simulink model "FaceDet_x4"  (Simulink 7.7)
settings: Solver=FixedStepDiscrete  StartTime=0  StopTime=10  RelTol=1e-3
libraries: simulink x257
(part 4 of 5)

== system FaceDet_x4/FaceDetection/FU/FeatureCalcMachine3/CalcFeatureVal ==
  note: Feature can't be bigger
      | than sfix18!!!
  Lines24x15 : Inport
  LineIdxs : Inport  Port=2
  NodeWeights : Inport  Port=3
  Add : Sum  OutDataTypeStr=sint(18)
  Conv0_s3 : DataTypeConversion  OutDataTypeStr=sint(3)
  Conv0_u8 : DataTypeConversion  OutDataTypeStr=uint8
  Conv1_s3 : DataTypeConversion  OutDataTypeStr=sint(3)
  Conv1_u8 : DataTypeConversion  OutDataTypeStr=uint8
  Conv2_s3 : DataTypeConversion  OutDataTypeStr=sint(3)
  Conv2_u8 : DataTypeConversion  OutDataTypeStr=uint8
  Conv3_s3 : DataTypeConversion  OutDataTypeStr=sint(3)
  Conv3_u8 : DataTypeConversion  OutDataTypeStr=uint8
  DivideBy4 : simulink/Logic and Bit Operations/Extract Bits  SystemSampleTime=-1  bitsToExtract=Range of bits  numBits=8  bitIdxRange=[0 17]  outScalingMode=Treat bit field as an integer
  FeatureAdder : Sum  Inputs=++++  OutDataTypeStr=sint(20)
  LineIdxDemux : Demux
  NodeWeightsDemux : Demux
  ProdWgt{0..3} (4 alike) : Product  OutDataTypeStr=sint(18)  RndMeth=Zero
  SelectLine{0..3} (4 alike) : Selector  IndexMode=Zero-based  IndexOptions=Index vector (port)  Indices=1  OutputSizes=1
  ColFeatureVal : Outport
  wires:
  ProdWgt0/1 -> FeatureAdder/1
  ProdWgt1/1 -> FeatureAdder/2
  Add/1 -> FeatureAdder/3
  ProdWgt3/1 -> FeatureAdder/4
  FeatureAdder/1 -> DivideBy4/1
  LineIdxDemux/1 -> Conv0_u8/1
  Conv0_u8/1 -> SelectLine0/2
  SelectLine0/1 -> ProdWgt0/1
  LineIdxDemux/2 -> Conv1_u8/1
  Conv1_u8/1 -> SelectLine1/2
  SelectLine1/1 -> ProdWgt1/1
  Conv2_u8/1 -> SelectLine2/2
  SelectLine2/1 -> ProdWgt2/1, Add/1
  LineIdxDemux/4 -> Conv3_u8/1
  Conv3_u8/1 -> SelectLine3/2
  SelectLine3/1 -> ProdWgt3/1
  Lines24x15/1 -> SelectLine2/1, SelectLine3/1, SelectLine1/1, SelectLine0/1
  LineIdxs/1 -> LineIdxDemux/1
  LineIdxDemux/3 -> Conv2_u8/1
  NodeWeights/1 -> NodeWeightsDemux/1
  NodeWeightsDemux/4 -> Conv3_s3/1
  NodeWeightsDemux/3 -> Conv2_s3/1
  NodeWeightsDemux/2 -> Conv1_s3/1
  NodeWeightsDemux/1 -> Conv0_s3/1
  Conv3_s3/1 -> ProdWgt3/2
  DivideBy4/1 -> ColFeatureVal/1
  Conv0_s3/1 -> ProdWgt0/2
  Conv1_s3/1 -> ProdWgt1/2
  Conv2_s3/1 -> ProdWgt2/2
  ProdWgt2/1 -> Add/2

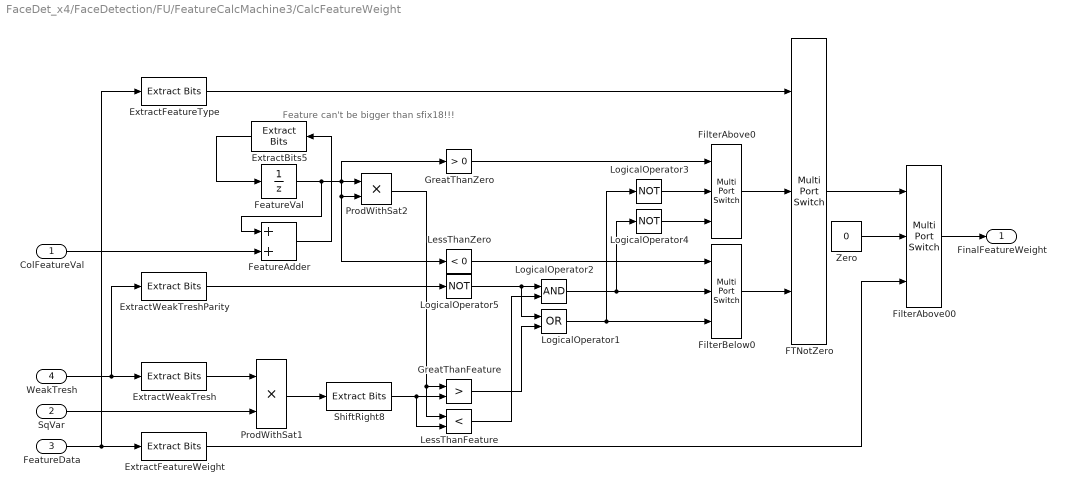
== system FaceDet_x4/FaceDetection/FU/FeatureCalcMachine3/CalcFeatureWeight ==
  note: Feature can't be bigger
      | than sfix18!!!
  ColFeatureVal : Inport
  SqVar : Inport  Port=2
  FeatureData : Inport  Port=3
  WeakTresh : Inport  Port=4
  ExtractBits5 : simulink/Logic and Bit Operations/Extract Bits  SystemSampleTime=-1  bitsToExtract=Range of bits  numBits=8  bitIdxRange=[0 17]  outScalingMode=Treat bit field as an integer
  ExtractFeatureType : simulink/Logic and Bit Operations/Extract Bits  SystemSampleTime=-1  bitsToExtract=Range of bits  numBits=8  bitIdxRange=[0 0]  outScalingMode=Treat bit field as an integer
  ExtractFeatureWeight : simulink/Logic and Bit Operations/Extract Bits  SystemSampleTime=-1  bitsToExtract=Range of bits  numBits=8  bitIdxRange=[1 16]  outScalingMode=Treat bit field as an integer
  ExtractWeakTresh : simulink/Logic and Bit Operations/Extract Bits  SystemSampleTime=-1  bitsToExtract=Range of bits  numBits=8  bitIdxRange=[1 24]  outScalingMode=Treat bit field as an integer
  ExtractWeakTreshParity : simulink/Logic and Bit Operations/Extract Bits  SystemSampleTime=-1  bitsToExtract=Range of bits  numBits=8  bitIdxRange=[0 0]  outScalingMode=Treat bit field as an integer
  FTNotZero : MultiPortSwitch  DataPortOrder=Zero-based contiguous  Inputs=2  zeroidx=on
  FeatureAdder : Sum  OutDataTypeStr=sint(19)
  FeatureVal : UnitDelay
  FilterAbove0 : MultiPortSwitch  DataPortOrder=Zero-based contiguous  Inputs=2  zeroidx=on
  FilterAbove00 : MultiPortSwitch  DataPortOrder=Zero-based contiguous  Inputs=2  zeroidx=on
  FilterBelow0 : MultiPortSwitch  DataPortOrder=Zero-based contiguous  Inputs=2  zeroidx=on
  GreatThanFeature : RelationalOperator  Operator=>  OutDataTypeStr=boolean
  GreatThanZero : simulink/Logic and Bit Operations/Compare To Zero  SystemSampleTime=-1  relop=>  LogicOutDataTypeMode=boolean  ZeroCross=off
  LessThanFeature : RelationalOperator  Operator=<  OutDataTypeStr=boolean
  LessThanZero : simulink/Logic and Bit Operations/Compare To Zero  SystemSampleTime=-1  relop=<  LogicOutDataTypeMode=boolean  ZeroCross=off
  LogicalOperator1 : Logic  Operator=OR  AllPortsSameDT=off  OutDataTypeStr=boolean
  LogicalOperator2 : Logic  AllPortsSameDT=off  OutDataTypeStr=boolean
  LogicalOperator3 : Logic  Operator=NOT  AllPortsSameDT=off  OutDataTypeStr=boolean
  LogicalOperator4 : Logic  Operator=NOT  AllPortsSameDT=off  OutDataTypeStr=boolean
  LogicalOperator5 : Logic  Operator=NOT  AllPortsSameDT=off  OutDataTypeStr=boolean
  ProdWithSat1 : Product  OutDataTypeStr=uint(32)  SaturateOnIntegerOverflow=on  RndMeth=Zero
  ProdWithSat2 : Product  OutDataTypeStr=uint32  SaturateOnIntegerOverflow=on  RndMeth=Zero
  ShiftRight8 : simulink/Logic and Bit Operations/Extract Bits  SystemSampleTime=-1  bitsToExtract=Range of bits  numBits=8  bitIdxRange=[8 31]  outScalingMode=Treat bit field as an integer
  Zero : Constant  Value=0  OutDataTypeStr=uint16
  FinalFeatureWeight : Outport
  wires:
  FeatureVal/1 -> FeatureAdder/1, GreatThanZero/1, ProdWithSat2/1, LessThanZero/1, ProdWithSat2/2
  FeatureAdder/1 -> ExtractBits5/1
  ProdWithSat2/1 -> GreatThanFeature/1, LessThanFeature/1
  LogicalOperator4/1 -> FilterAbove0/3
  ShiftRight8/1 -> LessThanFeature/2, GreatThanFeature/2
  ProdWithSat1/1 -> ShiftRight8/1
  FilterBelow0/1 -> FTNotZero/3
  FilterAbove0/1 -> FTNotZero/2
  LogicalOperator3/1 -> FilterAbove0/2
  GreatThanZero/1 -> FilterAbove0/1
  LessThanZero/1 -> FilterBelow0/1
  Zero/1 -> FilterAbove00/2
  FTNotZero/1 -> FilterAbove00/1
  LogicalOperator5/1 -> LogicalOperator2/1, LogicalOperator1/1
  LessThanFeature/1 -> LogicalOperator2/2
  LogicalOperator2/1 -> LogicalOperator4/1, FilterBelow0/2
  LogicalOperator1/1 -> LogicalOperator3/1, FilterBelow0/3
  GreatThanFeature/1 -> LogicalOperator1/2
  WeakTresh/1 -> ExtractWeakTresh/1, ExtractWeakTreshParity/1
  SqVar/1 -> ProdWithSat1/2
  FeatureData/1 -> ExtractFeatureWeight/1, ExtractFeatureType/1
  FilterAbove00/1 -> FinalFeatureWeight/1
  ColFeatureVal/1 -> FeatureAdder/2
  ExtractBits5/1 -> FeatureVal/1
  ExtractFeatureWeight/1 -> FilterAbove00/3
  ExtractFeatureType/1 -> FTNotZero/1
  ExtractWeakTresh/1 -> ProdWithSat1/1
  ExtractWeakTreshParity/1 -> LogicalOperator5/1

== system FaceDet_x4/FaceDetection/FU/MemBank/FeatureDataMem ==
  FeatureDataLatch : Inport
  FeatureDataExt : Inport  Port=2
  Comb4FeatureData : Mux
  FeatureData{0..3} (4 alike) : simulink/Additional Math & Discrete/Additional Discrete/Unit Delay Enabled  SystemSampleTime=-1  vinit=0  tsamp=-1
  FeatureData : Outport
  wires:
  FeatureDataExt/1 -> FeatureData0/1, FeatureData1/1, FeatureData2/1, FeatureData3/1
  FeatureData0/1 -> Comb4FeatureData/1
  FeatureDataLatch/1 -> FeatureData0/2, FeatureData1/2, FeatureData2/2, FeatureData3/2
  Comb4FeatureData/1 -> FeatureData/1
  FeatureData1/1 -> Comb4FeatureData/2
  FeatureData2/1 -> Comb4FeatureData/3
  FeatureData3/1 -> Comb4FeatureData/4

== system FaceDet_x4/FaceDetection/FU/MemBank/LineIdxsMem ==
  LineIdxsLatch : Inport
  LineIdxsExt : Inport  Port=2
  Comb4LineIdxs : Mux
  LineIdxsBank{0..3} (4 alike) : simulink/Additional Math & Discrete/Additional Discrete/Unit Delay Enabled  SystemSampleTime=-1  vinit=0  tsamp=-1
  LineIdxs : Outport
  wires:
  Comb4LineIdxs/1 -> LineIdxs/1
  LineIdxsLatch/1 -> LineIdxsBank0/2, LineIdxsBank1/2, LineIdxsBank2/2, LineIdxsBank3/2
  LineIdxsBank0/1 -> Comb4LineIdxs/1
  LineIdxsExt/1 -> LineIdxsBank0/1, LineIdxsBank1/1, LineIdxsBank2/1, LineIdxsBank3/1
  LineIdxsBank1/1 -> Comb4LineIdxs/2
  LineIdxsBank3/1 -> Comb4LineIdxs/4
  LineIdxsBank2/1 -> Comb4LineIdxs/3

== system FaceDet_x4/FaceDetection/FU/MemBank/NodeWeightsMem ==
  NodeWeightsCtrlRdAdr : Inport
  NodeWeightsCtrlWrAdr : Inport  Port=2
  NodeWeightsCtrlEn : Inport  Port=3
  NodeWeightsExt : Inport  Port=4
  Comb4NodeWeights : Mux
  NodeWeightsBank0 : Subsystem  mask(Dual-port RAM){ram_size=5}
      mask prompts: ram_size "Address port width (2 to 16)"
      mask help:
      | This block simulates a dual-port RAM with registered address.
      |
      | The read and write address port width is limited to between 2 to 16 bits.
      mask init:
      | hdlblkmask_dpram;
      settings: ErrorFcn=hdlblkmask_errfcn
      mask Help: helpview([docroot '/toolbox/slhdlcoder/slhdlcoder_ug.map'],'HDL_dual_port_RAM');
      mask Display: disp( 'DualPortRam' )
  NodeWeightsBank1 : Subsystem  mask(Dual-port RAM){ram_size=5}
      mask prompts: ram_size "Address port width (2 to 16)"
      mask help:
      | This block simulates a dual-port RAM with registered address.
      |
      | The read and write address port width is limited to between 2 to 16 bits.
      mask init:
      | hdlblkmask_dpram;
      settings: ErrorFcn=hdlblkmask_errfcn
      mask Help: helpview([docroot '/toolbox/slhdlcoder/slhdlcoder_ug.map'],'HDL_dual_port_RAM');
      mask Display: disp( 'DualPortRam' )
  NodeWeightsBank2 : Subsystem  mask(Dual-port RAM){ram_size=5}
      mask prompts: ram_size "Address port width (2 to 16)"
      mask help:
      | This block simulates a dual-port RAM with registered address.
      |
      | The read and write address port width is limited to between 2 to 16 bits.
      mask init:
      | hdlblkmask_dpram;
      settings: ErrorFcn=hdlblkmask_errfcn
      mask Help: helpview([docroot '/toolbox/slhdlcoder/slhdlcoder_ug.map'],'HDL_dual_port_RAM');
      mask Display: disp( 'DualPortRam' )
  NodeWeightsBank3 : Subsystem  mask(Dual-port RAM){ram_size=5}
      mask prompts: ram_size "Address port width (2 to 16)"
      mask help:
      | This block simulates a dual-port RAM with registered address.
      |
      | The read and write address port width is limited to between 2 to 16 bits.
      mask init:
      | hdlblkmask_dpram;
      settings: ErrorFcn=hdlblkmask_errfcn
      mask Help: helpview([docroot '/toolbox/slhdlcoder/slhdlcoder_ug.map'],'HDL_dual_port_RAM');
      mask Display: disp( 'DualPortRam' )
  NodeWeights : Outport
  wires:
  NodeWeightsExt/1 -> NodeWeightsBank0/2(wr_din), NodeWeightsBank2/2(wr_din), NodeWeightsBank3/2(wr_din), NodeWeightsBank1/2(wr_din)
  NodeWeightsBank3/1(rd_dout) -> Comb4NodeWeights/4
  NodeWeightsBank2/1(rd_dout) -> Comb4NodeWeights/3
  NodeWeightsBank1/1(rd_dout) -> Comb4NodeWeights/2
  NodeWeightsBank0/1(rd_dout) -> Comb4NodeWeights/1
  NodeWeightsCtrlWrAdr/1 -> NodeWeightsBank2/4(wr_addr), NodeWeightsBank3/4(wr_addr), NodeWeightsBank1/4(wr_addr), NodeWeightsBank0/4(wr_addr)
  NodeWeightsCtrlEn/1 -> NodeWeightsBank2/3(wr_en), NodeWeightsBank3/3(wr_en), NodeWeightsBank1/3(wr_en), NodeWeightsBank0/3(wr_en)
  NodeWeightsCtrlRdAdr/1 -> NodeWeightsBank2/1(rd_addr), NodeWeightsBank3/1(rd_addr), NodeWeightsBank1/1(rd_addr), NodeWeightsBank0/1(rd_addr)
  Comb4NodeWeights/1 -> NodeWeights/1

== system FaceDet_x4/FaceDetection/FU/MemBank/WeakTreshMem ==
  WeakTreshLatch : Inport
  WeakTreshExt : Inport  Port=2
  Comb4WeakTresh : Mux
  WeakTresh{0..3} (4 alike) : simulink/Additional Math & Discrete/Additional Discrete/Unit Delay Enabled  SystemSampleTime=-1  vinit=0  tsamp=-1
  WeakTresh : Outport
  wires:
  WeakTresh3/1 -> Comb4WeakTresh/4
  WeakTresh2/1 -> Comb4WeakTresh/3
  WeakTresh1/1 -> Comb4WeakTresh/2
  Comb4WeakTresh/1 -> WeakTresh/1
  WeakTreshLatch/1 -> WeakTresh2/2, WeakTresh3/2, WeakTresh1/2, WeakTresh0/2
  WeakTresh0/1 -> Comb4WeakTresh/1
  WeakTreshExt/1 -> WeakTresh2/1, WeakTresh3/1, WeakTresh1/1, WeakTresh0/1

== system FaceDet_x4/FaceDetection/FU/CalcIntegralImg/HorzRunningSum/Accumulator0 ==
  note: AccumulatorBlock
  In : Inport
  En : Inport  Port=2
  Rst : Inport  Port=3
  Adder : Sum  OutDataTypeStr=uint(NBits)
  UDlyER : Subsystem  mask(Unit Delay Enabled Resettable){vinit=0, tsamp=-1}
      mask prompts: vinit "Initial condition:"; tsamp "Sample time:"
      mask help:
      | Normally, the output is the signal u delayed by one sample period.
      | When the reset signal R is true, the state is always set equal to the initial condition parameter.  This reset action is vectorized and supports scalar expansion.
      | When the enable signal is false, the block is disabled, and the state and output values do not change except for resets.  The enable action is vectorized and supports scalar expansion.
      mask Display: dpoly(1,[1 0],'z')
  Acc : Outport
  wires:
  En/1 -> UDlyER/2(E)
  Rst/1 -> UDlyER/3(R)
  In/1 -> Adder/1
  Adder/1 -> UDlyER/1(u), Acc/1
  UDlyER/1(y) -> Adder/2

== system FaceDet_x4/FaceDetection/FU/CalcIntegralImg/HorzRunningSum/Accumulator1 ==
  note: AccumulatorBlock
  In : Inport
  En : Inport  Port=2
  Rst : Inport  Port=3
  Adder : Sum  OutDataTypeStr=uint(NBits)
  UDlyER : Subsystem  mask(Unit Delay Enabled Resettable){vinit=0, tsamp=-1}
      mask prompts: vinit "Initial condition:"; tsamp "Sample time:"
      mask help:
      | Normally, the output is the signal u delayed by one sample period.
      | When the reset signal R is true, the state is always set equal to the initial condition parameter.  This reset action is vectorized and supports scalar expansion.
      | When the enable signal is false, the block is disabled, and the state and output values do not change except for resets.  The enable action is vectorized and supports scalar expansion.
      mask Display: dpoly(1,[1 0],'z')
  Acc : Outport
  wires:
  UDlyER/1(y) -> Adder/2
  Adder/1 -> Acc/1, UDlyER/1(u)
  In/1 -> Adder/1
  Rst/1 -> UDlyER/3(R)
  En/1 -> UDlyER/2(E)

== system FaceDet_x4/FaceDetection/FU/CalcIntegralImg/HorzRunningSum/Accumulator10 ==
  note: AccumulatorBlock
  In : Inport
  En : Inport  Port=2
  Rst : Inport  Port=3
  Adder : Sum  OutDataTypeStr=uint(NBits)
  UDlyER : Subsystem  mask(Unit Delay Enabled Resettable){vinit=0, tsamp=-1}
      mask prompts: vinit "Initial condition:"; tsamp "Sample time:"
      mask help:
      | Normally, the output is the signal u delayed by one sample period.
      | When the reset signal R is true, the state is always set equal to the initial condition parameter.  This reset action is vectorized and supports scalar expansion.
      | When the enable signal is false, the block is disabled, and the state and output values do not change except for resets.  The enable action is vectorized and supports scalar expansion.
      mask Display: dpoly(1,[1 0],'z')
  Acc : Outport
  wires:
  En/1 -> UDlyER/2(E)
  Rst/1 -> UDlyER/3(R)
  In/1 -> Adder/1
  Adder/1 -> UDlyER/1(u), Acc/1
  UDlyER/1(y) -> Adder/2

== system FaceDet_x4/FaceDetection/FU/CalcIntegralImg/HorzRunningSum/Accumulator11 ==
  note: AccumulatorBlock
  In : Inport
  En : Inport  Port=2
  Rst : Inport  Port=3
  Adder : Sum  OutDataTypeStr=uint(NBits)
  UDlyER : Subsystem  mask(Unit Delay Enabled Resettable){vinit=0, tsamp=-1}
      mask prompts: vinit "Initial condition:"; tsamp "Sample time:"
      mask help:
      | Normally, the output is the signal u delayed by one sample period.
      | When the reset signal R is true, the state is always set equal to the initial condition parameter.  This reset action is vectorized and supports scalar expansion.
      | When the enable signal is false, the block is disabled, and the state and output values do not change except for resets.  The enable action is vectorized and supports scalar expansion.
      mask Display: dpoly(1,[1 0],'z')
  Acc : Outport
  wires:
  UDlyER/1(y) -> Adder/2
  Adder/1 -> Acc/1, UDlyER/1(u)
  In/1 -> Adder/1
  Rst/1 -> UDlyER/3(R)
  En/1 -> UDlyER/2(E)

== system FaceDet_x4/FaceDetection/FU/CalcIntegralImg/HorzRunningSum/Accumulator12 ==
  note: AccumulatorBlock
  In : Inport
  En : Inport  Port=2
  Rst : Inport  Port=3
  Adder : Sum  OutDataTypeStr=uint(NBits)
  UDlyER : Subsystem  mask(Unit Delay Enabled Resettable){vinit=0, tsamp=-1}
      mask prompts: vinit "Initial condition:"; tsamp "Sample time:"
      mask help:
      | Normally, the output is the signal u delayed by one sample period.
      | When the reset signal R is true, the state is always set equal to the initial condition parameter.  This reset action is vectorized and supports scalar expansion.
      | When the enable signal is false, the block is disabled, and the state and output values do not change except for resets.  The enable action is vectorized and supports scalar expansion.
      mask Display: dpoly(1,[1 0],'z')
  Acc : Outport
  wires:
  En/1 -> UDlyER/2(E)
  Rst/1 -> UDlyER/3(R)
  In/1 -> Adder/1
  Adder/1 -> UDlyER/1(u), Acc/1
  UDlyER/1(y) -> Adder/2

== system FaceDet_x4/FaceDetection/FU/CalcIntegralImg/HorzRunningSum/Accumulator13 ==
  note: AccumulatorBlock
  In : Inport
  En : Inport  Port=2
  Rst : Inport  Port=3
  Adder : Sum  OutDataTypeStr=uint(NBits)
  UDlyER : Subsystem  mask(Unit Delay Enabled Resettable){vinit=0, tsamp=-1}
      mask prompts: vinit "Initial condition:"; tsamp "Sample time:"
      mask help:
      | Normally, the output is the signal u delayed by one sample period.
      | When the reset signal R is true, the state is always set equal to the initial condition parameter.  This reset action is vectorized and supports scalar expansion.
      | When the enable signal is false, the block is disabled, and the state and output values do not change except for resets.  The enable action is vectorized and supports scalar expansion.
      mask Display: dpoly(1,[1 0],'z')
  Acc : Outport
  wires:
  UDlyER/1(y) -> Adder/2
  Adder/1 -> Acc/1, UDlyER/1(u)
  In/1 -> Adder/1
  Rst/1 -> UDlyER/3(R)
  En/1 -> UDlyER/2(E)

== system FaceDet_x4/FaceDetection/FU/CalcIntegralImg/HorzRunningSum/Accumulator14 ==
  note: AccumulatorBlock
  In : Inport
  En : Inport  Port=2
  Rst : Inport  Port=3
  Adder : Sum  OutDataTypeStr=uint(NBits)
  UDlyER : Subsystem  mask(Unit Delay Enabled Resettable){vinit=0, tsamp=-1}
      mask prompts: vinit "Initial condition:"; tsamp "Sample time:"
      mask help:
      | Normally, the output is the signal u delayed by one sample period.
      | When the reset signal R is true, the state is always set equal to the initial condition parameter.  This reset action is vectorized and supports scalar expansion.
      | When the enable signal is false, the block is disabled, and the state and output values do not change except for resets.  The enable action is vectorized and supports scalar expansion.
      mask Display: dpoly(1,[1 0],'z')
  Acc : Outport
  wires:
  En/1 -> UDlyER/2(E)
  Rst/1 -> UDlyER/3(R)
  In/1 -> Adder/1
  Adder/1 -> UDlyER/1(u), Acc/1
  UDlyER/1(y) -> Adder/2

== system FaceDet_x4/FaceDetection/FU/CalcIntegralImg/HorzRunningSum/Accumulator15 ==
  note: AccumulatorBlock
  In : Inport
  En : Inport  Port=2
  Rst : Inport  Port=3
  Adder : Sum  OutDataTypeStr=uint(NBits)
  UDlyER : Subsystem  mask(Unit Delay Enabled Resettable){vinit=0, tsamp=-1}
      mask prompts: vinit "Initial condition:"; tsamp "Sample time:"
      mask help:
      | Normally, the output is the signal u delayed by one sample period.
      | When the reset signal R is true, the state is always set equal to the initial condition parameter.  This reset action is vectorized and supports scalar expansion.
      | When the enable signal is false, the block is disabled, and the state and output values do not change except for resets.  The enable action is vectorized and supports scalar expansion.
      mask Display: dpoly(1,[1 0],'z')
  Acc : Outport
  wires:
  UDlyER/1(y) -> Adder/2
  Adder/1 -> Acc/1, UDlyER/1(u)
  In/1 -> Adder/1
  Rst/1 -> UDlyER/3(R)
  En/1 -> UDlyER/2(E)

== system FaceDet_x4/FaceDetection/FU/CalcIntegralImg/HorzRunningSum/Accumulator16 ==
  note: AccumulatorBlock
  In : Inport
  En : Inport  Port=2
  Rst : Inport  Port=3
  Adder : Sum  OutDataTypeStr=uint(NBits)
  UDlyER : Subsystem  mask(Unit Delay Enabled Resettable){vinit=0, tsamp=-1}
      mask prompts: vinit "Initial condition:"; tsamp "Sample time:"
      mask help:
      | Normally, the output is the signal u delayed by one sample period.
      | When the reset signal R is true, the state is always set equal to the initial condition parameter.  This reset action is vectorized and supports scalar expansion.
      | When the enable signal is false, the block is disabled, and the state and output values do not change except for resets.  The enable action is vectorized and supports scalar expansion.
      mask Display: dpoly(1,[1 0],'z')
  Acc : Outport
  wires:
  En/1 -> UDlyER/2(E)
  Rst/1 -> UDlyER/3(R)
  In/1 -> Adder/1
  Adder/1 -> UDlyER/1(u), Acc/1
  UDlyER/1(y) -> Adder/2

== system FaceDet_x4/FaceDetection/FU/CalcIntegralImg/HorzRunningSum/Accumulator17 ==
  note: AccumulatorBlock
  In : Inport
  En : Inport  Port=2
  Rst : Inport  Port=3
  Adder : Sum  OutDataTypeStr=uint(NBits)
  UDlyER : Subsystem  mask(Unit Delay Enabled Resettable){vinit=0, tsamp=-1}
      mask prompts: vinit "Initial condition:"; tsamp "Sample time:"
      mask help:
      | Normally, the output is the signal u delayed by one sample period.
      | When the reset signal R is true, the state is always set equal to the initial condition parameter.  This reset action is vectorized and supports scalar expansion.
      | When the enable signal is false, the block is disabled, and the state and output values do not change except for resets.  The enable action is vectorized and supports scalar expansion.
      mask Display: dpoly(1,[1 0],'z')
  Acc : Outport
  wires:
  UDlyER/1(y) -> Adder/2
  Adder/1 -> Acc/1, UDlyER/1(u)
  In/1 -> Adder/1
  Rst/1 -> UDlyER/3(R)
  En/1 -> UDlyER/2(E)

== system FaceDet_x4/FaceDetection/FU/CalcIntegralImg/HorzRunningSum/Accumulator18 ==
  note: AccumulatorBlock
  In : Inport
  En : Inport  Port=2
  Rst : Inport  Port=3
  Adder : Sum  OutDataTypeStr=uint(NBits)
  UDlyER : Subsystem  mask(Unit Delay Enabled Resettable){vinit=0, tsamp=-1}
      mask prompts: vinit "Initial condition:"; tsamp "Sample time:"
      mask help:
      | Normally, the output is the signal u delayed by one sample period.
      | When the reset signal R is true, the state is always set equal to the initial condition parameter.  This reset action is vectorized and supports scalar expansion.
      | When the enable signal is false, the block is disabled, and the state and output values do not change except for resets.  The enable action is vectorized and supports scalar expansion.
      mask Display: dpoly(1,[1 0],'z')
  Acc : Outport
  wires:
  En/1 -> UDlyER/2(E)
  Rst/1 -> UDlyER/3(R)
  In/1 -> Adder/1
  Adder/1 -> UDlyER/1(u), Acc/1
  UDlyER/1(y) -> Adder/2

== system FaceDet_x4/FaceDetection/FU/CalcIntegralImg/HorzRunningSum/Accumulator19 ==
  note: AccumulatorBlock
  In : Inport
  En : Inport  Port=2
  Rst : Inport  Port=3
  Adder : Sum  OutDataTypeStr=uint(NBits)
  UDlyER : Subsystem  mask(Unit Delay Enabled Resettable){vinit=0, tsamp=-1}
      mask prompts: vinit "Initial condition:"; tsamp "Sample time:"
      mask help:
      | Normally, the output is the signal u delayed by one sample period.
      | When the reset signal R is true, the state is always set equal to the initial condition parameter.  This reset action is vectorized and supports scalar expansion.
      | When the enable signal is false, the block is disabled, and the state and output values do not change except for resets.  The enable action is vectorized and supports scalar expansion.
      mask Display: dpoly(1,[1 0],'z')
  Acc : Outport
  wires:
  UDlyER/1(y) -> Adder/2
  Adder/1 -> Acc/1, UDlyER/1(u)
  In/1 -> Adder/1
  Rst/1 -> UDlyER/3(R)
  En/1 -> UDlyER/2(E)

== system FaceDet_x4/FaceDetection/FU/CalcIntegralImg/HorzRunningSum/Accumulator2 ==
  note: AccumulatorBlock
  In : Inport
  En : Inport  Port=2
  Rst : Inport  Port=3
  Adder : Sum  OutDataTypeStr=uint(NBits)
  UDlyER : Subsystem  mask(Unit Delay Enabled Resettable){vinit=0, tsamp=-1}
      mask prompts: vinit "Initial condition:"; tsamp "Sample time:"
      mask help:
      | Normally, the output is the signal u delayed by one sample period.
      | When the reset signal R is true, the state is always set equal to the initial condition parameter.  This reset action is vectorized and supports scalar expansion.
      | When the enable signal is false, the block is disabled, and the state and output values do not change except for resets.  The enable action is vectorized and supports scalar expansion.
      mask Display: dpoly(1,[1 0],'z')
  Acc : Outport
  wires:
  En/1 -> UDlyER/2(E)
  Rst/1 -> UDlyER/3(R)
  In/1 -> Adder/1
  Adder/1 -> UDlyER/1(u), Acc/1
  UDlyER/1(y) -> Adder/2

== system FaceDet_x4/FaceDetection/FU/CalcIntegralImg/HorzRunningSum/Accumulator20 ==
  note: AccumulatorBlock
  In : Inport
  En : Inport  Port=2
  Rst : Inport  Port=3
  Adder : Sum  OutDataTypeStr=uint(NBits)
  UDlyER : Subsystem  mask(Unit Delay Enabled Resettable){vinit=0, tsamp=-1}
      mask prompts: vinit "Initial condition:"; tsamp "Sample time:"
      mask help:
      | Normally, the output is the signal u delayed by one sample period.
      | When the reset signal R is true, the state is always set equal to the initial condition parameter.  This reset action is vectorized and supports scalar expansion.
      | When the enable signal is false, the block is disabled, and the state and output values do not change except for resets.  The enable action is vectorized and supports scalar expansion.
      mask Display: dpoly(1,[1 0],'z')
  Acc : Outport
  wires:
  En/1 -> UDlyER/2(E)
  Rst/1 -> UDlyER/3(R)
  In/1 -> Adder/1
  Adder/1 -> UDlyER/1(u), Acc/1
  UDlyER/1(y) -> Adder/2

== system FaceDet_x4/FaceDetection/FU/CalcIntegralImg/HorzRunningSum/Accumulator21 ==
  note: AccumulatorBlock
  In : Inport
  En : Inport  Port=2
  Rst : Inport  Port=3
  Adder : Sum  OutDataTypeStr=uint(NBits)
  UDlyER : Subsystem  mask(Unit Delay Enabled Resettable){vinit=0, tsamp=-1}
      mask prompts: vinit "Initial condition:"; tsamp "Sample time:"
      mask help:
      | Normally, the output is the signal u delayed by one sample period.
      | When the reset signal R is true, the state is always set equal to the initial condition parameter.  This reset action is vectorized and supports scalar expansion.
      | When the enable signal is false, the block is disabled, and the state and output values do not change except for resets.  The enable action is vectorized and supports scalar expansion.
      mask Display: dpoly(1,[1 0],'z')
  Acc : Outport
  wires:
  UDlyER/1(y) -> Adder/2
  Adder/1 -> Acc/1, UDlyER/1(u)
  In/1 -> Adder/1
  Rst/1 -> UDlyER/3(R)
  En/1 -> UDlyER/2(E)

== system FaceDet_x4/FaceDetection/FU/CalcIntegralImg/HorzRunningSum/Accumulator22 ==
  note: AccumulatorBlock
  In : Inport
  En : Inport  Port=2
  Rst : Inport  Port=3
  Adder : Sum  OutDataTypeStr=uint(NBits)
  UDlyER : Subsystem  mask(Unit Delay Enabled Resettable){vinit=0, tsamp=-1}
      mask prompts: vinit "Initial condition:"; tsamp "Sample time:"
      mask help:
      | Normally, the output is the signal u delayed by one sample period.
      | When the reset signal R is true, the state is always set equal to the initial condition parameter.  This reset action is vectorized and supports scalar expansion.
      | When the enable signal is false, the block is disabled, and the state and output values do not change except for resets.  The enable action is vectorized and supports scalar expansion.
      mask Display: dpoly(1,[1 0],'z')
  Acc : Outport
  wires:
  En/1 -> UDlyER/2(E)
  Rst/1 -> UDlyER/3(R)
  In/1 -> Adder/1
  Adder/1 -> UDlyER/1(u), Acc/1
  UDlyER/1(y) -> Adder/2

== system FaceDet_x4/FaceDetection/FU/CalcIntegralImg/HorzRunningSum/Accumulator23 ==
  note: AccumulatorBlock
  In : Inport
  En : Inport  Port=2
  Rst : Inport  Port=3
  Adder : Sum  OutDataTypeStr=uint(NBits)
  UDlyER : Subsystem  mask(Unit Delay Enabled Resettable){vinit=0, tsamp=-1}
      mask prompts: vinit "Initial condition:"; tsamp "Sample time:"
      mask help:
      | Normally, the output is the signal u delayed by one sample period.
      | When the reset signal R is true, the state is always set equal to the initial condition parameter.  This reset action is vectorized and supports scalar expansion.
      | When the enable signal is false, the block is disabled, and the state and output values do not change except for resets.  The enable action is vectorized and supports scalar expansion.
      mask Display: dpoly(1,[1 0],'z')
  Acc : Outport
  wires:
  UDlyER/1(y) -> Adder/2
  Adder/1 -> Acc/1, UDlyER/1(u)
  In/1 -> Adder/1
  Rst/1 -> UDlyER/3(R)
  En/1 -> UDlyER/2(E)

== system FaceDet_x4/FaceDetection/FU/CalcIntegralImg/HorzRunningSum/Accumulator3 ==
  note: AccumulatorBlock
  In : Inport
  En : Inport  Port=2
  Rst : Inport  Port=3
  Adder : Sum  OutDataTypeStr=uint(NBits)
  UDlyER : Subsystem  mask(Unit Delay Enabled Resettable){vinit=0, tsamp=-1}
      mask prompts: vinit "Initial condition:"; tsamp "Sample time:"
      mask help:
      | Normally, the output is the signal u delayed by one sample period.
      | When the reset signal R is true, the state is always set equal to the initial condition parameter.  This reset action is vectorized and supports scalar expansion.
      | When the enable signal is false, the block is disabled, and the state and output values do not change except for resets.  The enable action is vectorized and supports scalar expansion.
      mask Display: dpoly(1,[1 0],'z')
  Acc : Outport
  wires:
  UDlyER/1(y) -> Adder/2
  Adder/1 -> Acc/1, UDlyER/1(u)
  In/1 -> Adder/1
  Rst/1 -> UDlyER/3(R)
  En/1 -> UDlyER/2(E)

== system FaceDet_x4/FaceDetection/FU/CalcIntegralImg/HorzRunningSum/Accumulator4 ==
  note: AccumulatorBlock
  In : Inport
  En : Inport  Port=2
  Rst : Inport  Port=3
  Adder : Sum  OutDataTypeStr=uint(NBits)
  UDlyER : Subsystem  mask(Unit Delay Enabled Resettable){vinit=0, tsamp=-1}
      mask prompts: vinit "Initial condition:"; tsamp "Sample time:"
      mask help:
      | Normally, the output is the signal u delayed by one sample period.
      | When the reset signal R is true, the state is always set equal to the initial condition parameter.  This reset action is vectorized and supports scalar expansion.
      | When the enable signal is false, the block is disabled, and the state and output values do not change except for resets.  The enable action is vectorized and supports scalar expansion.
      mask Display: dpoly(1,[1 0],'z')
  Acc : Outport
  wires:
  En/1 -> UDlyER/2(E)
  Rst/1 -> UDlyER/3(R)
  In/1 -> Adder/1
  Adder/1 -> UDlyER/1(u), Acc/1
  UDlyER/1(y) -> Adder/2

== system FaceDet_x4/FaceDetection/FU/CalcIntegralImg/HorzRunningSum/Accumulator5 ==
  note: AccumulatorBlock
  In : Inport
  En : Inport  Port=2
  Rst : Inport  Port=3
  Adder : Sum  OutDataTypeStr=uint(NBits)
  UDlyER : Subsystem  mask(Unit Delay Enabled Resettable){vinit=0, tsamp=-1}
      mask prompts: vinit "Initial condition:"; tsamp "Sample time:"
      mask help:
      | Normally, the output is the signal u delayed by one sample period.
      | When the reset signal R is true, the state is always set equal to the initial condition parameter.  This reset action is vectorized and supports scalar expansion.
      | When the enable signal is false, the block is disabled, and the state and output values do not change except for resets.  The enable action is vectorized and supports scalar expansion.
      mask Display: dpoly(1,[1 0],'z')
  Acc : Outport
  wires:
  UDlyER/1(y) -> Adder/2
  Adder/1 -> Acc/1, UDlyER/1(u)
  In/1 -> Adder/1
  Rst/1 -> UDlyER/3(R)
  En/1 -> UDlyER/2(E)

== system FaceDet_x4/FaceDetection/FU/CalcIntegralImg/HorzRunningSum/Accumulator6 ==
  note: AccumulatorBlock
  In : Inport
  En : Inport  Port=2
  Rst : Inport  Port=3
  Adder : Sum  OutDataTypeStr=uint(NBits)
  UDlyER : Subsystem  mask(Unit Delay Enabled Resettable){vinit=0, tsamp=-1}
      mask prompts: vinit "Initial condition:"; tsamp "Sample time:"
      mask help:
      | Normally, the output is the signal u delayed by one sample period.
      | When the reset signal R is true, the state is always set equal to the initial condition parameter.  This reset action is vectorized and supports scalar expansion.
      | When the enable signal is false, the block is disabled, and the state and output values do not change except for resets.  The enable action is vectorized and supports scalar expansion.
      mask Display: dpoly(1,[1 0],'z')
  Acc : Outport
  wires:
  En/1 -> UDlyER/2(E)
  Rst/1 -> UDlyER/3(R)
  In/1 -> Adder/1
  Adder/1 -> UDlyER/1(u), Acc/1
  UDlyER/1(y) -> Adder/2

== system FaceDet_x4/FaceDetection/FU/CalcIntegralImg/HorzRunningSum/Accumulator7 ==
  note: AccumulatorBlock
  In : Inport
  En : Inport  Port=2
  Rst : Inport  Port=3
  Adder : Sum  OutDataTypeStr=uint(NBits)
  UDlyER : Subsystem  mask(Unit Delay Enabled Resettable){vinit=0, tsamp=-1}
      mask prompts: vinit "Initial condition:"; tsamp "Sample time:"
      mask help:
      | Normally, the output is the signal u delayed by one sample period.
      | When the reset signal R is true, the state is always set equal to the initial condition parameter.  This reset action is vectorized and supports scalar expansion.
      | When the enable signal is false, the block is disabled, and the state and output values do not change except for resets.  The enable action is vectorized and supports scalar expansion.
      mask Display: dpoly(1,[1 0],'z')
  Acc : Outport
  wires:
  UDlyER/1(y) -> Adder/2
  Adder/1 -> Acc/1, UDlyER/1(u)
  In/1 -> Adder/1
  Rst/1 -> UDlyER/3(R)
  En/1 -> UDlyER/2(E)

== system FaceDet_x4/FaceDetection/FU/CalcIntegralImg/HorzRunningSum/Accumulator8 ==
  note: AccumulatorBlock
  In : Inport
  En : Inport  Port=2
  Rst : Inport  Port=3
  Adder : Sum  OutDataTypeStr=uint(NBits)
  UDlyER : Subsystem  mask(Unit Delay Enabled Resettable){vinit=0, tsamp=-1}
      mask prompts: vinit "Initial condition:"; tsamp "Sample time:"
      mask help:
      | Normally, the output is the signal u delayed by one sample period.
      | When the reset signal R is true, the state is always set equal to the initial condition parameter.  This reset action is vectorized and supports scalar expansion.
      | When the enable signal is false, the block is disabled, and the state and output values do not change except for resets.  The enable action is vectorized and supports scalar expansion.
      mask Display: dpoly(1,[1 0],'z')
  Acc : Outport
  wires:
  En/1 -> UDlyER/2(E)
  Rst/1 -> UDlyER/3(R)
  In/1 -> Adder/1
  Adder/1 -> UDlyER/1(u), Acc/1
  UDlyER/1(y) -> Adder/2

== system FaceDet_x4/FaceDetection/FU/CalcIntegralImg/HorzRunningSum/Accumulator9 ==
  note: AccumulatorBlock
  In : Inport
  En : Inport  Port=2
  Rst : Inport  Port=3
  Adder : Sum  OutDataTypeStr=uint(NBits)
  UDlyER : Subsystem  mask(Unit Delay Enabled Resettable){vinit=0, tsamp=-1}
      mask prompts: vinit "Initial condition:"; tsamp "Sample time:"
      mask help:
      | Normally, the output is the signal u delayed by one sample period.
      | When the reset signal R is true, the state is always set equal to the initial condition parameter.  This reset action is vectorized and supports scalar expansion.
      | When the enable signal is false, the block is disabled, and the state and output values do not change except for resets.  The enable action is vectorized and supports scalar expansion.
      mask Display: dpoly(1,[1 0],'z')
  Acc : Outport
  wires:
  UDlyER/1(y) -> Adder/2
  Adder/1 -> Acc/1, UDlyER/1(u)
  In/1 -> Adder/1
  Rst/1 -> UDlyER/3(R)
  En/1 -> UDlyER/2(E)

== system FaceDet_x4/FaceDetection/FU/CalcIntegralImg/VerticalSum/IntgImg1 ==
  In1 : Inport
  In2 : Inport  Port=2
  In3 : Inport  Port=3
  In4 : Inport  Port=4
  In5 : Inport  Port=5
  Sum : Sum  OutDataTypeStr=uint(11)
  Sum1 : Sum  OutDataTypeStr=uint(12)
  Sum2 : Sum  OutDataTypeStr=uint(12)
  Sum3 : Sum  OutDataTypeStr=uint(12)
  Out1 : Outport
  Out2 : Outport  Port=2
  Out3 : Outport  Port=3
  Out4 : Outport  Port=4
  Out5 : Outport  Port=5
  wires:
  Sum/1 -> Sum1/1, Out2/1
  In1/1 -> Sum/1, Out1/1
  In2/1 -> Sum/2
  In3/1 -> Sum1/2
  Sum2/1 -> Sum3/1, Out4/1
  Sum1/1 -> Sum2/1, Out3/1
  In4/1 -> Sum2/2
  In5/1 -> Sum3/2
  Sum3/1 -> Out5/1

== system FaceDet_x4/FaceDetection/FU/CalcIntegralImg/VerticalSum/IntgImg2 ==
  In1 : Inport
  In2 : Inport  Port=2
  In3 : Inport  Port=3
  In4 : Inport  Port=4
  In5 : Inport  Port=5
  Sum : Sum  OutDataTypeStr=uint(12)
  Sum1 : Sum  OutDataTypeStr=uint(13)
  Sum2 : Sum  OutDataTypeStr=uint(13)
  Sum3 : Sum  OutDataTypeStr=uint(13)
  Out1 : Outport
  Out2 : Outport  Port=2
  Out3 : Outport  Port=3
  Out4 : Outport  Port=4
  Out5 : Outport  Port=5
  wires:
  Sum3/1 -> Out5/1
  In5/1 -> Sum3/2
  In4/1 -> Sum2/2
  Sum1/1 -> Out3/1, Sum2/1
  Sum2/1 -> Out4/1, Sum3/1
  In3/1 -> Sum1/2
  In2/1 -> Sum/2
  In1/1 -> Out1/1, Sum/1
  Sum/1 -> Out2/1, Sum1/1

== system FaceDet_x4/FaceDetection/FU/CalcIntegralImg/VerticalSum/IntgImg3 ==
  In1 : Inport
  In2 : Inport  Port=2
  In3 : Inport  Port=3
  In4 : Inport  Port=4
  In5 : Inport  Port=5
  Sum : Sum  OutDataTypeStr=uint(13)
  Sum1 : Sum  OutDataTypeStr=uint(13)
  Sum2 : Sum  OutDataTypeStr=uint(14)
  Sum3 : Sum  OutDataTypeStr=uint(14)
  Out1 : Outport
  Out2 : Outport  Port=2
  Out3 : Outport  Port=3
  Out4 : Outport  Port=4
  Out5 : Outport  Port=5
  wires:
  Sum3/1 -> Out5/1
  In5/1 -> Sum3/2
  In4/1 -> Sum2/2
  Sum1/1 -> Out3/1, Sum2/1
  Sum2/1 -> Out4/1, Sum3/1
  In3/1 -> Sum1/2
  In2/1 -> Sum/2
  In1/1 -> Out1/1, Sum/1
  Sum/1 -> Out2/1, Sum1/1

== system FaceDet_x4/FaceDetection/FU/CalcIntegralImg/VerticalSum/IntgImg4 ==
  In1 : Inport
  In2 : Inport  Port=2
  In3 : Inport  Port=3
  In4 : Inport  Port=4
  In5 : Inport  Port=5
  Sum{,1..3} (4 alike) : Sum  OutDataTypeStr=uint(14)
  Out1 : Outport
  Out2 : Outport  Port=2
  Out3 : Outport  Port=3
  Out4 : Outport  Port=4
  Out5 : Outport  Port=5
  wires:
  Sum3/1 -> Out5/1
  In5/1 -> Sum3/2
  In4/1 -> Sum2/2
  Sum1/1 -> Out3/1, Sum2/1
  Sum2/1 -> Out4/1, Sum3/1
  In3/1 -> Sum1/2
  In2/1 -> Sum/2
  In1/1 -> Out1/1, Sum/1
  Sum/1 -> Out2/1, Sum1/1

== system FaceDet_x4/FaceDetection/FU/CalcIntegralImg/VerticalSum/IntgImg5 ==
  In1 : Inport
  In2 : Inport  Port=2
  In3 : Inport  Port=3
  In4 : Inport  Port=4
  In5 : Inport  Port=5
  Sum{,1..3} (4 alike) : Sum  OutDataTypeStr=uint(14)
  Out1 : Outport
  Out2 : Outport  Port=2
  Out3 : Outport  Port=3
  Out4 : Outport  Port=4
  Out5 : Outport  Port=5
  wires:
  Sum3/1 -> Out5/1
  In5/1 -> Sum3/2
  In4/1 -> Sum2/2
  Sum1/1 -> Out3/1, Sum2/1
  Sum2/1 -> Out4/1, Sum3/1
  In3/1 -> Sum1/2
  In2/1 -> Sum/2
  In1/1 -> Out1/1, Sum/1
  Sum/1 -> Out2/1, Sum1/1

== system FaceDet_x4/FaceDetection/FU/CalcIntegralImg/VerticalSum/IntgImg6 ==
  In1 : Inport
  In2 : Inport  Port=2
  In3 : Inport  Port=3
  In4 : Inport  Port=4
  Sum : Sum  OutDataTypeStr=uint(15)
  Sum1 : Sum  OutDataTypeStr=uint(15)
  Sum2 : Sum  OutDataTypeStr=uint(15)
  Out1 : Outport
  Out2 : Outport  Port=2
  Out3 : Outport  Port=3
  Out4 : Outport  Port=4
  wires:
  In4/1 -> Sum2/2
  Sum1/1 -> Out3/1, Sum2/1
  Sum2/1 -> Out4/1
  In3/1 -> Sum1/2
  In2/1 -> Sum/2
  In1/1 -> Out1/1, Sum/1
  Sum/1 -> Out2/1, Sum1/1

== system FaceDet_x4/FaceDetection/FU/CalcNNVariance/AccVar/UDlyER ==
  note: UnitDelayEnabledResettable
  u : Inport
  E : Inport  Port=2
  R : Inport  Port=3
  FixPt Unit Delay1 : UnitDelay  X0=vinit  SampleTime=tsamp
  ICond : Constant  Value=vinit  OutDataTypeStr=Inherit: Inherit via back propagation
  SwitchEn : MultiPortSwitch  DataPortOrder=Zero-based contiguous  Inputs=2  zeroidx=on
  SwitchRst : MultiPortSwitch  DataPortOrder=Zero-based contiguous  Inputs=2  zeroidx=on
  y : Outport
  wires:
  R/1 -> SwitchRst/1  "Reset"
  SwitchEn/1 -> SwitchRst/2
  u/1 -> SwitchEn/3  "Data"
  E/1 -> SwitchEn/1  "Enable"
  FixPt Unit Delay1/1 -> y/1, SwitchEn/2  "Xold"
  SwitchRst/1 -> FixPt Unit Delay1/1  "Xnew"
  ICond/1 -> SwitchRst/3  "IVal"

== system FaceDet_x4/FaceDetection/FU/CalcNNVariance/CounterModulo2/UDlyER ==
  note: UnitDelayEnabledResettable
  u : Inport
  E : Inport  Port=2
  R : Inport  Port=3
  FixPt Unit Delay1 : UnitDelay  X0=vinit  SampleTime=tsamp
  ICond : Constant  Value=vinit  OutDataTypeStr=Inherit: Inherit via back propagation
  SwitchEn : MultiPortSwitch  DataPortOrder=Zero-based contiguous  Inputs=2  zeroidx=on
  SwitchRst : MultiPortSwitch  DataPortOrder=Zero-based contiguous  Inputs=2  zeroidx=on
  y : Outport
  wires:
  ICond/1 -> SwitchRst/3  "IVal"
  SwitchRst/1 -> FixPt Unit Delay1/1  "Xnew"
  FixPt Unit Delay1/1 -> SwitchEn/2, y/1  "Xold"
  E/1 -> SwitchEn/1  "Enable"
  u/1 -> SwitchEn/3  "Data"
  SwitchEn/1 -> SwitchRst/2
  R/1 -> SwitchRst/1  "Reset"

== system FaceDet_x4/FaceDetection/FU/MemBank/NodeWeightsMem/NodeWeightsBank0 ==
  rd_addr : Inport
  wr_din : Inport  Port=2
  wr_en : Inport  Port=3  OutDataTypeStr=boolean
  wr_addr : Inport  Port=4
  convert : DataTypeConversion  OutDataTypeStr=uint16
  convert1 : DataTypeConversion  OutDataTypeStr=uint16
  ram : UnitDelay
  rd_addr_d : UnitDelay
  select : Selector  IndexMode=Zero-based  InputPortWidth=2^ram_size  IndexOptions=Index vector (port)  Indices=[1 3]  OutputSizes=1
  switch : Switch  Criteria=u2 ~= 0
  wr_port : Assignment  IndexMode=Zero-based  IndexOptions=Index vector (port)  Indices=1  OutputSizes=[1 1]
  rd_dout : Outport
  wires:
  wr_port/1 -> switch/1
  switch/1 -> ram/1
  ram/1 -> wr_port/1, select/1, switch/3
  wr_din/1 -> wr_port/2
  wr_en/1 -> switch/2
  wr_addr/1 -> convert/1
  rd_addr/1 -> rd_addr_d/1
  select/1 -> rd_dout/1
  convert/1 -> wr_port/3
  convert1/1 -> select/2
  rd_addr_d/1 -> convert1/1

== system FaceDet_x4/FaceDetection/FU/MemBank/NodeWeightsMem/NodeWeightsBank1 ==
  rd_addr : Inport
  wr_din : Inport  Port=2
  wr_en : Inport  Port=3  OutDataTypeStr=boolean
  wr_addr : Inport  Port=4
  convert : DataTypeConversion  OutDataTypeStr=uint16
  convert1 : DataTypeConversion  OutDataTypeStr=uint16
  ram : UnitDelay
  rd_addr_d : UnitDelay
  select : Selector  IndexMode=Zero-based  InputPortWidth=2^ram_size  IndexOptions=Index vector (port)  Indices=[1 3]  OutputSizes=1
  switch : Switch  Criteria=u2 ~= 0
  wr_port : Assignment  IndexMode=Zero-based  IndexOptions=Index vector (port)  Indices=1  OutputSizes=[1 1]
  rd_dout : Outport
  wires:
  rd_addr_d/1 -> convert1/1
  convert1/1 -> select/2
  convert/1 -> wr_port/3
  select/1 -> rd_dout/1
  rd_addr/1 -> rd_addr_d/1
  wr_addr/1 -> convert/1
  wr_en/1 -> switch/2
  wr_din/1 -> wr_port/2
  ram/1 -> switch/3, select/1, wr_port/1
  switch/1 -> ram/1
  wr_port/1 -> switch/1

== system FaceDet_x4/FaceDetection/FU/MemBank/NodeWeightsMem/NodeWeightsBank2 ==
  rd_addr : Inport
  wr_din : Inport  Port=2
  wr_en : Inport  Port=3  OutDataTypeStr=boolean
  wr_addr : Inport  Port=4
  convert : DataTypeConversion  OutDataTypeStr=uint16
  convert1 : DataTypeConversion  OutDataTypeStr=uint16
  ram : UnitDelay
  rd_addr_d : UnitDelay
  select : Selector  IndexMode=Zero-based  InputPortWidth=2^ram_size  IndexOptions=Index vector (port)  Indices=[1 3]  OutputSizes=1
  switch : Switch  Criteria=u2 ~= 0
  wr_port : Assignment  IndexMode=Zero-based  IndexOptions=Index vector (port)  Indices=1  OutputSizes=[1 1]
  rd_dout : Outport
  wires:
  wr_port/1 -> switch/1
  switch/1 -> ram/1
  ram/1 -> wr_port/1, select/1, switch/3
  wr_din/1 -> wr_port/2
  wr_en/1 -> switch/2
  wr_addr/1 -> convert/1
  rd_addr/1 -> rd_addr_d/1
  select/1 -> rd_dout/1
  convert/1 -> wr_port/3
  convert1/1 -> select/2
  rd_addr_d/1 -> convert1/1

== system FaceDet_x4/FaceDetection/FU/MemBank/NodeWeightsMem/NodeWeightsBank3 ==
  rd_addr : Inport
  wr_din : Inport  Port=2
  wr_en : Inport  Port=3  OutDataTypeStr=boolean
  wr_addr : Inport  Port=4
  convert : DataTypeConversion  OutDataTypeStr=uint16
  convert1 : DataTypeConversion  OutDataTypeStr=uint16
  ram : UnitDelay
  rd_addr_d : UnitDelay
  select : Selector  IndexMode=Zero-based  InputPortWidth=2^ram_size  IndexOptions=Index vector (port)  Indices=[1 3]  OutputSizes=1
  switch : Switch  Criteria=u2 ~= 0
  wr_port : Assignment  IndexMode=Zero-based  IndexOptions=Index vector (port)  Indices=1  OutputSizes=[1 1]
  rd_dout : Outport
  wires:
  rd_addr_d/1 -> convert1/1
  convert1/1 -> select/2
  convert/1 -> wr_port/3
  select/1 -> rd_dout/1
  rd_addr/1 -> rd_addr_d/1
  wr_addr/1 -> convert/1
  wr_en/1 -> switch/2
  wr_din/1 -> wr_port/2
  ram/1 -> switch/3, select/1, wr_port/1
  switch/1 -> ram/1
  wr_port/1 -> switch/1

== system FaceDet_x4/FaceDetection/FU/CalcIntegralImg/HorzRunningSum/Accumulator0/UDlyER ==
  note: UnitDelayEnabledResettable
  u : Inport
  E : Inport  Port=2
  R : Inport  Port=3
  FixPt Unit Delay1 : UnitDelay  X0=vinit  SampleTime=tsamp
  ICond : Constant  Value=vinit  OutDataTypeStr=Inherit: Inherit via back propagation
  SwitchEn : MultiPortSwitch  DataPortOrder=Zero-based contiguous  Inputs=2  zeroidx=on
  SwitchRst : MultiPortSwitch  DataPortOrder=Zero-based contiguous  Inputs=2  zeroidx=on
  y : Outport
  wires:
  ICond/1 -> SwitchRst/3  "IVal"
  SwitchRst/1 -> FixPt Unit Delay1/1  "Xnew"
  FixPt Unit Delay1/1 -> SwitchEn/2, y/1  "Xold"
  E/1 -> SwitchEn/1  "Enable"
  u/1 -> SwitchEn/3  "Data"
  SwitchEn/1 -> SwitchRst/2
  R/1 -> SwitchRst/1  "Reset"

== system FaceDet_x4/FaceDetection/FU/CalcIntegralImg/HorzRunningSum/Accumulator1/UDlyER ==
  note: UnitDelayEnabledResettable
  u : Inport
  E : Inport  Port=2
  R : Inport  Port=3
  FixPt Unit Delay1 : UnitDelay  X0=vinit  SampleTime=tsamp
  ICond : Constant  Value=vinit  OutDataTypeStr=Inherit: Inherit via back propagation
  SwitchEn : MultiPortSwitch  DataPortOrder=Zero-based contiguous  Inputs=2  zeroidx=on
  SwitchRst : MultiPortSwitch  DataPortOrder=Zero-based contiguous  Inputs=2  zeroidx=on
  y : Outport
  wires:
  R/1 -> SwitchRst/1  "Reset"
  SwitchEn/1 -> SwitchRst/2
  u/1 -> SwitchEn/3  "Data"
  E/1 -> SwitchEn/1  "Enable"
  FixPt Unit Delay1/1 -> y/1, SwitchEn/2  "Xold"
  SwitchRst/1 -> FixPt Unit Delay1/1  "Xnew"
  ICond/1 -> SwitchRst/3  "IVal"

== system FaceDet_x4/FaceDetection/FU/CalcIntegralImg/HorzRunningSum/Accumulator10/UDlyER ==
  note: UnitDelayEnabledResettable
  u : Inport
  E : Inport  Port=2
  R : Inport  Port=3
  FixPt Unit Delay1 : UnitDelay  X0=vinit  SampleTime=tsamp
  ICond : Constant  Value=vinit  OutDataTypeStr=Inherit: Inherit via back propagation
  SwitchEn : MultiPortSwitch  DataPortOrder=Zero-based contiguous  Inputs=2  zeroidx=on
  SwitchRst : MultiPortSwitch  DataPortOrder=Zero-based contiguous  Inputs=2  zeroidx=on
  y : Outport
  wires:
  ICond/1 -> SwitchRst/3  "IVal"
  SwitchRst/1 -> FixPt Unit Delay1/1  "Xnew"
  FixPt Unit Delay1/1 -> SwitchEn/2, y/1  "Xold"
  E/1 -> SwitchEn/1  "Enable"
  u/1 -> SwitchEn/3  "Data"
  SwitchEn/1 -> SwitchRst/2
  R/1 -> SwitchRst/1  "Reset"

== system FaceDet_x4/FaceDetection/FU/CalcIntegralImg/HorzRunningSum/Accumulator11/UDlyER ==
  note: UnitDelayEnabledResettable
  u : Inport
  E : Inport  Port=2
  R : Inport  Port=3
  FixPt Unit Delay1 : UnitDelay  X0=vinit  SampleTime=tsamp
  ICond : Constant  Value=vinit  OutDataTypeStr=Inherit: Inherit via back propagation
  SwitchEn : MultiPortSwitch  DataPortOrder=Zero-based contiguous  Inputs=2  zeroidx=on
  SwitchRst : MultiPortSwitch  DataPortOrder=Zero-based contiguous  Inputs=2  zeroidx=on
  y : Outport
  wires:
  R/1 -> SwitchRst/1  "Reset"
  SwitchEn/1 -> SwitchRst/2
  u/1 -> SwitchEn/3  "Data"
  E/1 -> SwitchEn/1  "Enable"
  FixPt Unit Delay1/1 -> y/1, SwitchEn/2  "Xold"
  SwitchRst/1 -> FixPt Unit Delay1/1  "Xnew"
  ICond/1 -> SwitchRst/3  "IVal"

== system FaceDet_x4/FaceDetection/FU/CalcIntegralImg/HorzRunningSum/Accumulator12/UDlyER ==
  note: UnitDelayEnabledResettable
  u : Inport
  E : Inport  Port=2
  R : Inport  Port=3
  FixPt Unit Delay1 : UnitDelay  X0=vinit  SampleTime=tsamp
  ICond : Constant  Value=vinit  OutDataTypeStr=Inherit: Inherit via back propagation
  SwitchEn : MultiPortSwitch  DataPortOrder=Zero-based contiguous  Inputs=2  zeroidx=on
  SwitchRst : MultiPortSwitch  DataPortOrder=Zero-based contiguous  Inputs=2  zeroidx=on
  y : Outport
  wires:
  ICond/1 -> SwitchRst/3  "IVal"
  SwitchRst/1 -> FixPt Unit Delay1/1  "Xnew"
  FixPt Unit Delay1/1 -> SwitchEn/2, y/1  "Xold"
  E/1 -> SwitchEn/1  "Enable"
  u/1 -> SwitchEn/3  "Data"
  SwitchEn/1 -> SwitchRst/2
  R/1 -> SwitchRst/1  "Reset"

== system FaceDet_x4/FaceDetection/FU/CalcIntegralImg/HorzRunningSum/Accumulator13/UDlyER ==
  note: UnitDelayEnabledResettable
  u : Inport
  E : Inport  Port=2
  R : Inport  Port=3
  FixPt Unit Delay1 : UnitDelay  X0=vinit  SampleTime=tsamp
  ICond : Constant  Value=vinit  OutDataTypeStr=Inherit: Inherit via back propagation
  SwitchEn : MultiPortSwitch  DataPortOrder=Zero-based contiguous  Inputs=2  zeroidx=on
  SwitchRst : MultiPortSwitch  DataPortOrder=Zero-based contiguous  Inputs=2  zeroidx=on
  y : Outport
  wires:
  R/1 -> SwitchRst/1  "Reset"
  SwitchEn/1 -> SwitchRst/2
  u/1 -> SwitchEn/3  "Data"
  E/1 -> SwitchEn/1  "Enable"
  FixPt Unit Delay1/1 -> y/1, SwitchEn/2  "Xold"
  SwitchRst/1 -> FixPt Unit Delay1/1  "Xnew"
  ICond/1 -> SwitchRst/3  "IVal"

== system FaceDet_x4/FaceDetection/FU/CalcIntegralImg/HorzRunningSum/Accumulator14/UDlyER ==
  note: UnitDelayEnabledResettable
  u : Inport
  E : Inport  Port=2
  R : Inport  Port=3
  FixPt Unit Delay1 : UnitDelay  X0=vinit  SampleTime=tsamp
  ICond : Constant  Value=vinit  OutDataTypeStr=Inherit: Inherit via back propagation
  SwitchEn : MultiPortSwitch  DataPortOrder=Zero-based contiguous  Inputs=2  zeroidx=on
  SwitchRst : MultiPortSwitch  DataPortOrder=Zero-based contiguous  Inputs=2  zeroidx=on
  y : Outport
  wires:
  ICond/1 -> SwitchRst/3  "IVal"
  SwitchRst/1 -> FixPt Unit Delay1/1  "Xnew"
  FixPt Unit Delay1/1 -> SwitchEn/2, y/1  "Xold"
  E/1 -> SwitchEn/1  "Enable"
  u/1 -> SwitchEn/3  "Data"
  SwitchEn/1 -> SwitchRst/2
  R/1 -> SwitchRst/1  "Reset"
